simulink model "singleJointDiagram"  (R2021b)
settings: Solver=VariableStepAuto  StartTime=0.0  StopTime=10.0  RelTol=1e-3
values from neighbouring files (symbols this model uses):
  Joint = 1/(s+1)    [build_Simulink_diagram.m]
  Kaw = Ki_p    (= 1)    [build_Simulink_diagram.m]
  Ki_p = 1    [build_Simulink_diagram.m]
  Kp_p = 1    [build_Simulink_diagram.m]
  Kp_v = 1    [build_Simulink_diagram.m]
  Tfu = 1/70    (= 0.0142857142857)    [build_Simulink_diagram.m]
libraries: simulink x2, eeGeneralControl x1
settings Model: Creator=monti  LastModifiedBy=miche

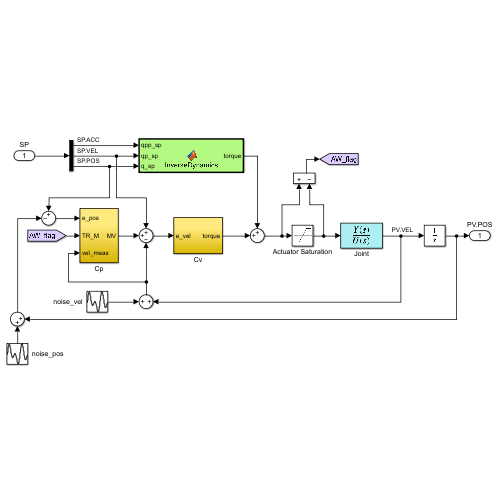
[thumbnail: Simulink's stored preview of the top-level diagram]
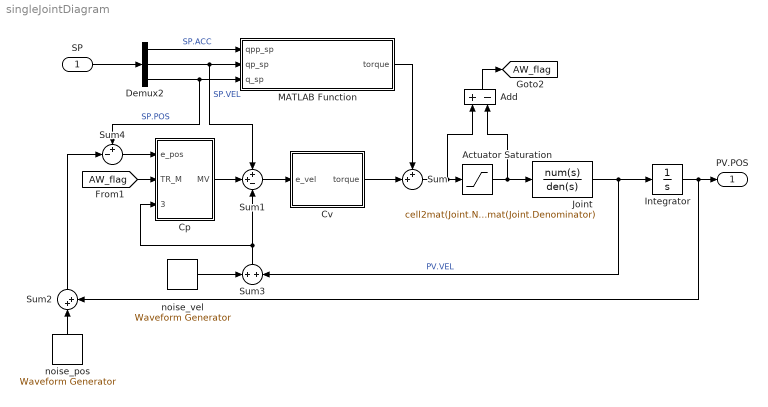
== system singleJointDiagram ==
  SP : Inport
  Actuator Saturation : Saturate  UpperLimit=150  LowerLimit=-150
  Add : Sum  Inputs=+-
  Cp : Subsystem
  Cv : Subsystem
  Demux2 : Demux  Outputs=3
  Integrator : Integrator
  Joint : TransferFcn  Tag=Giunto  Numerator=cell2mat(Joint.Numerator)  Denominator=cell2mat(Joint.Denominator)
  MATLAB Function : MATLAB Function  TreatAsAtomicUnit=on
  Sum : Sum  Inputs=++|
  Sum1 : Sum  Inputs=++-
  Sum2 : Sum  Inputs=|++
  Sum3 : Sum  Inputs=+|+
  Sum4 : Sum  Inputs=+-|
  noise_pos : simulink/Sources/Waveform Generator  OutMin=[]  OutMax=[]  OutDataTypeStr=double  SelectedSignal=1  BlockNames=MultiportSwitch_e3df3653d217406  SampleTime=0.1
  noise_vel : simulink/Sources/Waveform Generator  OutMin=[]  OutMax=[]  OutDataTypeStr=double  SelectedSignal=1  BlockNames=MultiportSwitch_e3df3653d217406  SampleTime=0.1
  PV.POS : Outport
  tag scope: AW_flag=global
  wires:
  Cp/1(MV) -> Sum1/2
  Sum3/1 -> Sum1/3, Cp/3(vel_meas)
  noise_pos/1 -> Sum2/1
  SP/1 -> Demux2/1
  MATLAB Function/1(torque) -> Sum/1
  Integrator/1 -> Sum2/2, PV.POS/1
  Demux2/2 -> MATLAB Function/2(qp_sp), Sum1/1  "SP.VEL"
  Demux2/1 -> MATLAB Function/1(qpp_sp)  "SP.ACC"
  Joint/1 -> Sum3/2, Integrator/1  "PV.VEL"
  noise_vel/1 -> Sum3/1
  Sum/1 -> Add/1, Actuator Saturation/1
  Demux2/3 -> MATLAB Function/3(q_sp), Sum4/1  "SP.POS"
  Actuator Saturation/1 -> Joint/1, Add/2
  Add/1 -> [AW_flag]
  [AW_flag] -> Cp/2(TR_M)
  Sum4/1 -> Cp/1(e_pos)
  Sum2/1 -> Sum4/2
  Sum1/1 -> Cv/1(e_vel)
  Cv/1(torque) -> Sum/2

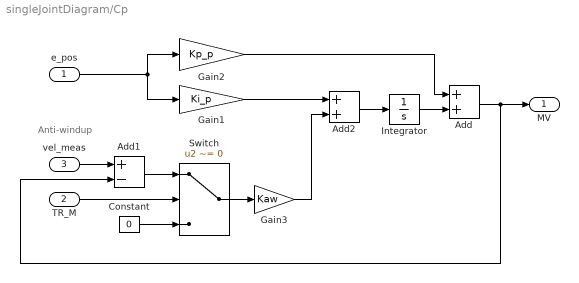
== system singleJointDiagram/Cp ==
  note: Anti-windup
  e_pos : Inport
  TR_M : Inport  Port=2
  vel_meas : Inport  Port=3
  Add : Sum
  Add1 : Sum  Inputs=+-
  Add2 : Sum
  Constant : Constant  Value=0
  Gain1 : Gain  Gain=Ki_p
  Gain2 : Gain  Gain=Kp_p
  Gain3 : Gain  Gain=Kaw
  Integrator : Integrator
  Switch : Switch  Criteria=u2 ~= 0
  MV : Outport
  wires:
  Constant/1 -> Switch/3
  vel_meas/1 -> Add1/1
  Add1/1 -> Switch/1
  TR_M/1 -> Switch/2
  e_pos/1 -> Gain2/1, Gain1/1
  Gain2/1 -> Add/1
  Add2/1 -> Integrator/1
  Integrator/1 -> Add/2
  Switch/1 -> Gain3/1
  Add/1 -> Add1/2, MV/1
  Gain1/1 -> Add2/1
  Gain3/1 -> Add2/2

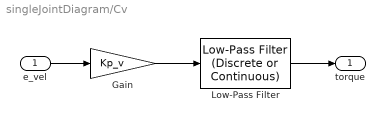
== system singleJointDiagram/Cv ==
  e_vel : Inport
  Gain : Gain  Gain=Kp_v
  Low-Pass Filter : eeGeneralControl/Low-Pass Filter (Discrete or Continuous)  K=1  T=Tfu  B=inf  A=-inf  init_option=Specify as parameter  x0=0  Ts=0
  torque : Outport
  wires:
  e_vel/1 -> Gain/1
  Gain/1 -> Low-Pass Filter/1
  Low-Pass Filter/1 -> torque/1

== matlab function singleJointDiagram/MATLAB Function ==
  data: qpp_sp input; torque output; qp_sp input; q_sp input
function torque = InverseDynamics(qpp_sp,qp_sp,q_sp)

FFW = SP;
